simulink model "PlatooningUsingV2VTestBench"  (R2025a)
settings: Solver=ode23tb  StartTime=0.0  StopTime=stopTime  RelTol=1e-1  AbsTol=5e-5
PostLoadFcn:
  | helperSLPlatooningUsingV2VSetup
InitFcn:
  | figureName = 'Platooning Simulation Results';
  | hFig = findobj('Type','Figure','Name',figureName);
  | close(hFig)
values from neighbouring files (symbols this model uses):
  L = vehicleDimension.TractorLength + vehicleDimension.TrailerLength + vehicleDimension.InterConnection - vehicleDimension.Overlap + spacing    [helperSLPlatooningUsingV2VSetup.m]
  spacing = 7    [helperSLPlatooningUsingV2VSetup.m]
undefined symbols (not defined in the file or in its folder): accelerationProfile, C1, DiscIntNeverNeededParam, initialActorPose, K1, K2, N, sceneOrigin, Sim3dSensor, tractor, Ts, Tsv, vehicleDimension
libraries: simulink x7, sim3dautolib x6, slpidlib x2, sim3dcameralib x1, sim3dlib x1, visionsinks x1
(part 1 of 2)
CloseFcn:
  | helperSLPlatooningUsingV2VCleanup
settings Model: SimulationMode=accelerator  Creator=The MathWorks, Inc.  LastModifiedBy=The MathWorks, Inc.
settings SolverCC: SolverJacobianMethodControl=FullPerturbation  ZeroCrossAlgorithm=Adaptive  DecoupledContinuousIntegration=on  MinimalZcImpactIntegration=on  MaxZcPerStep=1.0
settings OptimizationCC: ReuseModelBlockBuffer=off
settings DebuggingCC: IgnoredZcDiagnostic=none  UnconnectedInputMsg=warning  UnconnectedOutputMsg=warning  UnconnectedLineMsg=warning  SubsystemReferenceDiagnosticForUnitTest=warning
settings ModelReferenceCC: EnableRefExpFcnMdlSchedulingChecks=on
settings RTWCC: GPUComputeCapability=3.5  DLArmComputeVersion=19.05

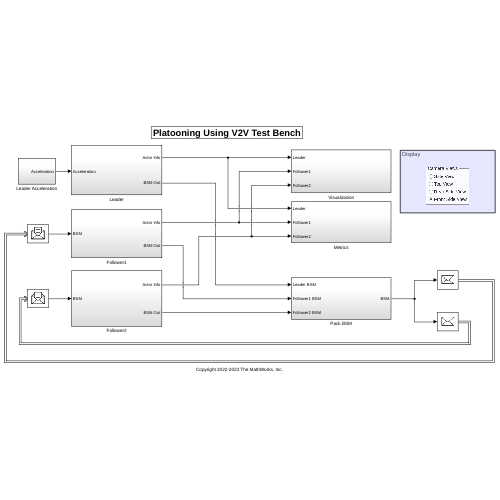
[thumbnail: Simulink's stored preview of the top-level diagram]
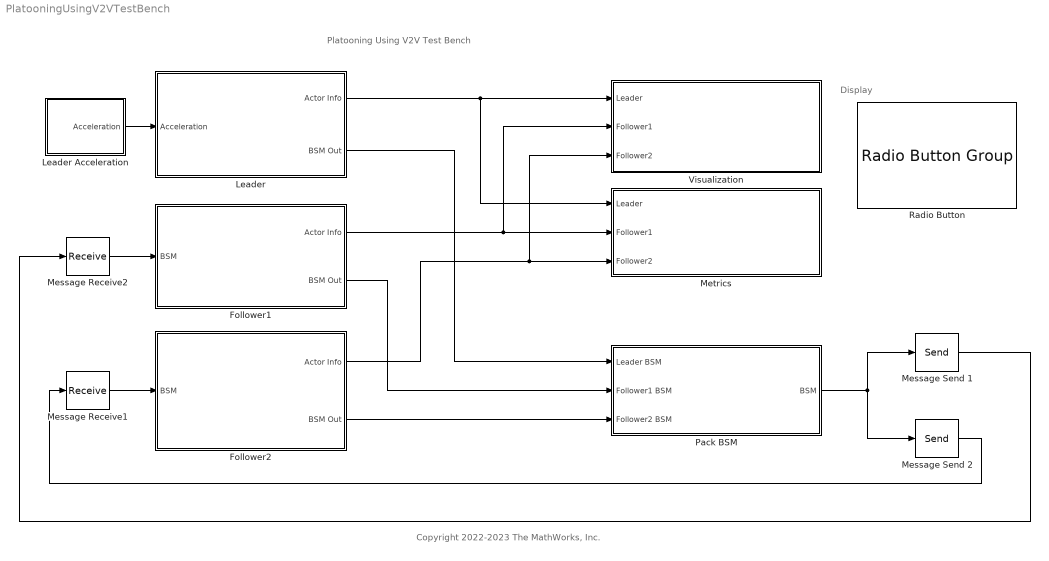
== system PlatooningUsingV2VTestBench ==
  note: Display
  note: Platooning Using V2V Test Bench
  note: Copyright 2022-2023 The MathWorks, Inc.
  Follower1 : Subsystem
  Follower2 : Subsystem
  Leader : Subsystem
  Leader Acceleration : Subsystem
  Message Receive1 : Receive  InputPortMessageModes=m  UseInternalQueue=off  SampleTime=Ts
  Message Receive2 : Receive  InputPortMessageModes=m  UseInternalQueue=off  SampleTime=Ts
  Message Send 1 : Send  OutputPortMessageModes=m
  Message Send 2 : Send  OutputPortMessageModes=m
  Metrics : Subsystem
  Pack BSM : Subsystem
  Radio Button : RadioButtonGroup  LabelPosition=Hide  SelectedLabel=Front Side View  ButtonGroupName=Camera Views
  Visualization : Subsystem
  wires:
  Leader Acceleration/1(Acceleration) -> Leader/1(Acceleration)
  Message Receive1/1 -> Follower2/1(BSM)
  Message Receive2/1 -> Follower1/1(BSM)
  Pack BSM/1(BSM) -> Message Send 2/1, Message Send 1/1
  Follower2/2(BSM Out) -> Pack BSM/3(Follower2 BSM)
  Follower1/2(BSM Out) -> Pack BSM/2(Follower1 BSM)
  Leader/2(BSM Out) -> Pack BSM/1(Leader BSM)
  Leader/1(Actor Info) -> Visualization/1(Leader), Metrics/1(Leader)
  Follower1/1(Actor Info) -> Metrics/2(Follower1), Visualization/2(Follower1)
  Follower2/1(Actor Info) -> Metrics/3(Follower2), Visualization/3(Follower2)
  Message Send 2/1 -> Message Receive1/1
  Message Send 1/1 -> Message Receive2/1

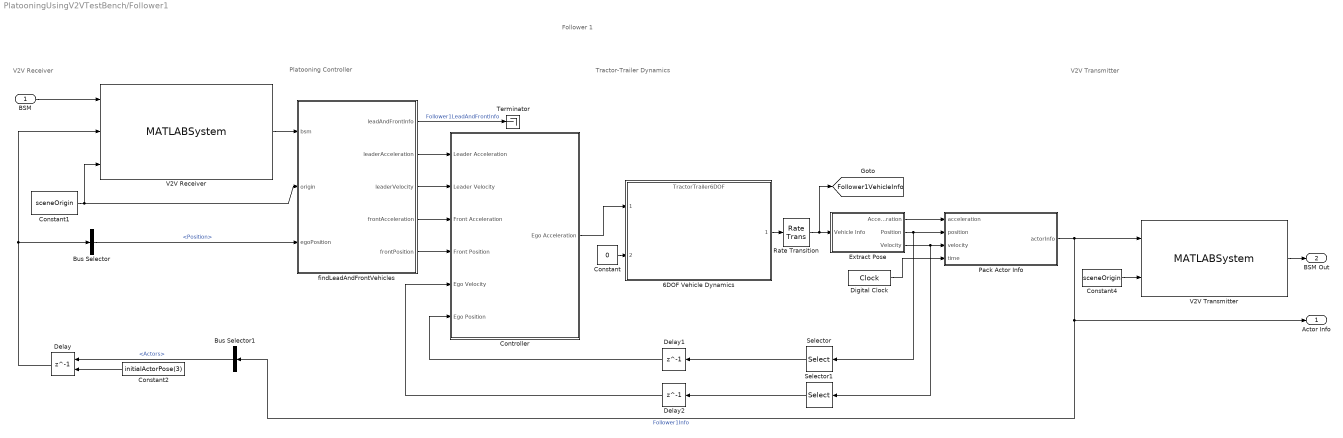
== system PlatooningUsingV2VTestBench/Follower1 ==
  note: V2V Transmitter
  note: Follower 1
  note: Tractor-Trailer Dynamics
  note: Platooning Controller
  note: V2V Receiver
  BSM : Inport
  6DOF Vehicle Dynamics : ModelReference  ModelNameDialog=TractorTrailer6DOF.slx  UsingDefaultArgumentValue=0,0,0,0,0,0,0,0  ModelReferenceVersion=5.2  initialTractorPosition=initialActorPose(3).Position  initialTractorVelocity=initialActorPose(3).Velocity  initialTractorOrientation=[0 0 0]  initialTractorRotationRates=[0 0 0]  initialTrailerPosition=initialActorPose(4).Position  initialTrailerVelocity=initialActorPose(4).Velocity  initialTrailerOrientation=[0 0 0]  initialTrailerRotationRates=[0 0 0]
  Bus Selector : BusSelector  OutputSignals=Position
  Bus Selector1 : BusSelector  OutputSignals=Actors
  Constant : Constant  Value=0  SampleTime=Ts
  Constant1 : Constant  Value=sceneOrigin  SampleTime=Ts
  Constant2 : Constant  Value=initialActorPose(3)  OutDataTypeStr=Bus: BusActorPose  SampleTime=-1
  Constant4 : Constant  Value=sceneOrigin  SampleTime=Ts
  Controller : Subsystem
  Delay : Delay  DelayLength=1  InitialConditionSource=Input port  SampleTime=Ts
      settings: InputPortMap=u0,p4
  Delay1 : Delay  DelayLength=1  InitialCondition=initialActorPose(3).Position(1)
  Delay2 : Delay  DelayLength=1  InitialCondition=initialActorPose(3).Velocity(1)
  Digital Clock : DigitalClock  SampleTime=Ts
  Extract Pose : Subsystem
  Pack Actor Info : MATLAB Function  TreatAsAtomicUnit=on  mask{initialActorInfo=initialActorPose(3), outputStruct=Simulink.Bus.createMATLABStruct('BusActorsInfo')}
      mask prompts: initialActorInfo "Initial Actor Info"; outputStruct "Output Struct"
  Rate Transition : RateTransition  OutPortSampleTime=Ts
  Selector : Selector  InputPortWidth=3  IndexOptions=Index vector (dialog)  Indices=1  OutputSizes=1
  Selector1 : Selector  InputPortWidth=3  IndexOptions=Index vector (dialog)  Indices=1  OutputSizes=1
  Terminator : Terminator
  V2V Receiver : MATLABSystem  System=HelperV2VReceiver  SnrCurves=channelAttributes  OutputStruct=Simulink.Bus.createMATLABStruct('BusBSM')  SimulateUsing=Code generation
      mask Type: HelperV2VReceiver
  V2V Transmitter : MATLABSystem  System=HelperV2VTransmitter  SampleTime=Ts  OutputStruct=Simulink.Bus.createMATLABStruct('BusBSM')  SimulateUsing=Code generation
      mask Type: HelperV2VTransmitter
  findLeadAndFrontVehicles : MATLAB Function  TreatAsAtomicUnit=on  mask(Process BSM data){egoID=initialActorPose(3).ActorID, outputStruct=Simulink.Bus.createMATLABStruct('BusLeadAndFrontInfo')}
      mask prompts: egoID "Actor ID"; outputStruct "Output Struct"
      mask help: Convert the BSM input data into physical values and generates object detection reports for the inputs to the multiObjectTracker
  Actor Info : Outport
  BSM Out : Outport  Port=2
  tag scope: Follower1VehicleInfo=global
  wires:
  Controller/1("Ego Acceleration ") -> 6DOF Vehicle Dynamics/1
  BSM/1 -> V2V Receiver/1
  Constant1/1 -> V2V Receiver/3, findLeadAndFrontVehicles/2(origin)
  Constant2/1 -> Delay/2
  Delay/1 -> Bus Selector/1, V2V Receiver/2
  V2V Receiver/1 -> findLeadAndFrontVehicles/1(bsm)
  Delay1/1 -> Controller/6("Ego Position ")
  Delay2/1 -> Controller/5("Ego Velocity ")
  6DOF Vehicle Dynamics/1 -> Rate Transition/1
  Bus Selector/1 -> findLeadAndFrontVehicles/3(egoPosition)  "<Position>"
  findLeadAndFrontVehicles/2(leaderAcceleration) -> Controller/1(Leader Acceleration)
  findLeadAndFrontVehicles/3(leaderVelocity) -> Controller/2("Leader Velocity ")
  findLeadAndFrontVehicles/4(frontAcceleration) -> Controller/3("Front Acceleration ")
  findLeadAndFrontVehicles/5(frontPosition) -> Controller/4("Front Position ")
  Constant/1 -> 6DOF Vehicle Dynamics/2
  Rate Transition/1 -> Extract Pose/1(Vehicle Info), [Follower1VehicleInfo]
  Extract Pose/1(Acceleration) -> Pack Actor Info/1(acceleration)
  Extract Pose/2(Position) -> Selector/1, Pack Actor Info/2(position)
  Extract Pose/3(Velocity) -> Selector1/1, Pack Actor Info/3(velocity)
  Selector/1 -> Delay1/1
  Selector1/1 -> Delay2/1
  findLeadAndFrontVehicles/1(leadAndFrontInfo) -> Terminator/1  "Follower1LeadAndFrontInfo"
  V2V Transmitter/1 -> BSM Out/1
  Constant4/1 -> V2V Transmitter/2
  Pack Actor Info/1(actorInfo) -> V2V Transmitter/1, Actor Info/1, Bus Selector1/1  "Follower1Info"
  Digital Clock/1 -> Pack Actor Info/4(time)
  Bus Selector1/1 -> Delay/1  "<Actors>"

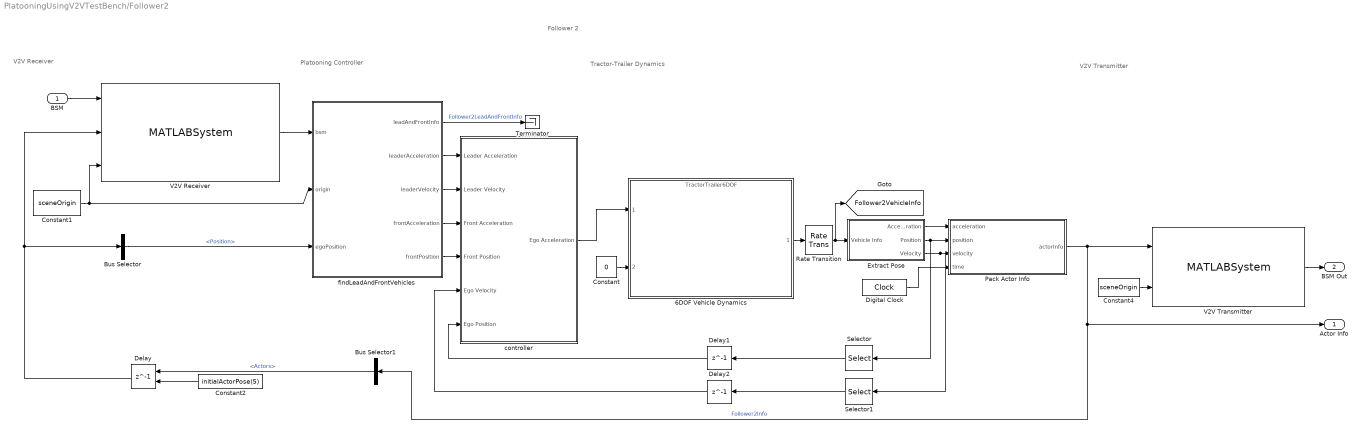
== system PlatooningUsingV2VTestBench/Follower2 ==
  note: V2V Receiver
  note: Follower 2
  note: Tractor-Trailer Dynamics
  note: Platooning Controller
  note: V2V Transmitter
  BSM : Inport
  6DOF Vehicle Dynamics : ModelReference  ModelNameDialog=TractorTrailer6DOF.slx  UsingDefaultArgumentValue=0,0,0,0,0,0,0,0  ModelReferenceVersion=5.2  initialTractorPosition=initialActorPose(5).Position  initialTractorVelocity=initialActorPose(5).Velocity  initialTractorOrientation=[0 0 0]  initialTractorRotationRates=[0 0 0]  initialTrailerPosition=initialActorPose(6).Position  initialTrailerVelocity=initialActorPose(6).Velocity  initialTrailerOrientation=[0 0 0]  initialTrailerRotationRates=[0 0 0]
  Bus Selector : BusSelector  OutputSignals=Position
  Bus Selector1 : BusSelector  OutputSignals=Actors
  Constant : Constant  Value=0  SampleTime=Ts
  Constant1 : Constant  Value=sceneOrigin  SampleTime=Ts
  Constant2 : Constant  Value=initialActorPose(5)  OutDataTypeStr=Bus: BusActorPose  SampleTime=-1
  Constant4 : Constant  Value=sceneOrigin  SampleTime=Ts
  Delay : Delay  DelayLength=1  InitialConditionSource=Input port  SampleTime=Ts
      settings: InputPortMap=u0,p4
  Delay1 : Delay  DelayLength=1  InitialCondition=initialActorPose(5).Position(1)
  Delay2 : Delay  DelayLength=1  InitialCondition=initialActorPose(5).Velocity(1)
  Digital Clock : DigitalClock  SampleTime=Ts
  Extract Pose : Subsystem
  Pack Actor Info : MATLAB Function  TreatAsAtomicUnit=on  mask{initialActorInfo=initialActorPose(5), outputStruct=Simulink.Bus.createMATLABStruct('BusActorsInfo')}
      mask prompts: initialActorInfo "Initial Actor Info"; outputStruct "Output Struct"
  Rate Transition : RateTransition  OutPortSampleTime=Ts
  Selector : Selector  InputPortWidth=3  IndexOptions=Index vector (dialog)  Indices=1  OutputSizes=1
  Selector1 : Selector  InputPortWidth=3  IndexOptions=Index vector (dialog)  Indices=1  OutputSizes=1
  Terminator : Terminator
  V2V Receiver : MATLABSystem  System=HelperV2VReceiver  SnrCurves=channelAttributes  OutputStruct=Simulink.Bus.createMATLABStruct('BusBSM')  SimulateUsing=Code generation
      mask Type: HelperV2VReceiver
  V2V Transmitter : MATLABSystem  System=HelperV2VTransmitter  SampleTime=Ts  OutputStruct=Simulink.Bus.createMATLABStruct('BusBSM')  SimulateUsing=Code generation
      mask Type: HelperV2VTransmitter
  controller : Subsystem
  findLeadAndFrontVehicles : MATLAB Function  TreatAsAtomicUnit=on  mask(Process BSM data){egoID=initialActorPose(5).ActorID, outputStruct=Simulink.Bus.createMATLABStruct('BusLeadAndFrontInfo')}
      mask prompts: egoID "Actor ID"; outputStruct "Output Struct"
      mask help: Convert the BSM input data into physical values and generates object detection reports for the inputs to the multiObjectTracker
  Actor Info : Outport
  BSM Out : Outport  Port=2
  tag scope: Follower2VehicleInfo=global
  wires:
  findLeadAndFrontVehicles/5(frontPosition) -> controller/4("Front Position ")
  findLeadAndFrontVehicles/3(leaderVelocity) -> controller/2(Leader Velocity)
  findLeadAndFrontVehicles/2(leaderAcceleration) -> controller/1(Leader Acceleration)
  BSM/1 -> V2V Receiver/1
  V2V Receiver/1 -> findLeadAndFrontVehicles/1(bsm)
  findLeadAndFrontVehicles/4(frontAcceleration) -> controller/3("Front Acceleration ")
  Constant1/1 -> V2V Receiver/3, findLeadAndFrontVehicles/2(origin)
  Constant2/1 -> Delay/2
  Delay/1 -> V2V Receiver/2, Bus Selector/1
  controller/1("Ego Acceleration ") -> 6DOF Vehicle Dynamics/1
  Delay1/1 -> controller/6(Ego Position)
  Delay2/1 -> controller/5("Ego Velocity ")
  6DOF Vehicle Dynamics/1 -> Rate Transition/1
  Bus Selector/1 -> findLeadAndFrontVehicles/3(egoPosition)  "<Position>"
  Extract Pose/1(Acceleration) -> Pack Actor Info/1(acceleration)
  Constant/1 -> 6DOF Vehicle Dynamics/2
  Rate Transition/1 -> Extract Pose/1(Vehicle Info), [Follower2VehicleInfo]
  Extract Pose/2(Position) -> Pack Actor Info/2(position), Selector/1
  Extract Pose/3(Velocity) -> Selector1/1, Pack Actor Info/3(velocity)
  Selector/1 -> Delay1/1
  Selector1/1 -> Delay2/1
  findLeadAndFrontVehicles/1(leadAndFrontInfo) -> Terminator/1  "Follower2LeadAndFrontInfo"
  Constant4/1 -> V2V Transmitter/2
  Pack Actor Info/1(actorInfo) -> V2V Transmitter/1, Actor Info/1, Bus Selector1/1  "Follower2Info"
  V2V Transmitter/1 -> BSM Out/1
  Digital Clock/1 -> Pack Actor Info/4(time)
  Bus Selector1/1 -> Delay/1  "<Actors>"

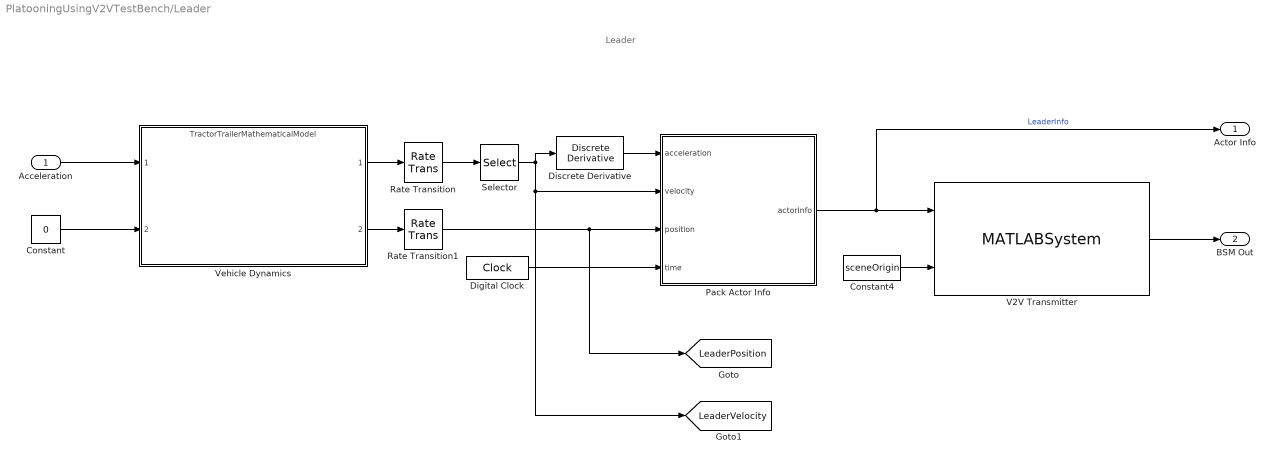
== system PlatooningUsingV2VTestBench/Leader ==
  note: Leader
  Acceleration : Inport
  Constant : Constant  Value=0
  Constant4 : Constant  Value=sceneOrigin  SampleTime=Ts
  Digital Clock : DigitalClock  SampleTime=Ts
  Discrete Derivative : simulink/Discrete/Discrete Derivative  gainval=1.0  ICPrevScaledInput=0.0  OutMin=[]  OutMax=[]  OutDataType=fixdt(1, 16)  OutScaling=2^-10  DoSatur=off
  Pack Actor Info : MATLAB Function  TreatAsAtomicUnit=on  mask{initialActorInfo=initialActorPose(1), outputStruct=Simulink.Bus.createMATLABStruct('BusActorsInfo')}
      mask prompts: initialActorInfo "Initial Actor Info"; outputStruct "Output Struct"
  Rate Transition : RateTransition  OutPortSampleTime=Ts
  Rate Transition1 : RateTransition  OutPortSampleTime=Ts
  Selector : Selector  InputPortWidth=8  IndexOptions=Index vector (dialog)  Indices=[1 2]  OutputSizes=1
  V2V Transmitter : MATLABSystem  System=HelperV2VTransmitter  SampleTime=Ts  OutputStruct=Simulink.Bus.createMATLABStruct('BusBSM')  SimulateUsing=Code generation
      mask Type: HelperV2VTransmitter
  Vehicle Dynamics : ModelReference  ModelNameDialog=TractorTrailerMathematicalModel.slx  UsingDefaultArgumentValue=0,0,0,0  SimulationMode=Normal  ModelReferenceVersion=3.0  initialPosition=initialActorPose(1).Position  initialVelocity=initialActorPose(1).Velocity  theta=0  beta=0
  Actor Info : Outport
  BSM Out : Outport  Port=2
  tag scope: LeaderPosition=global, LeaderVelocity=global
  wires:
  Vehicle Dynamics/1 -> Rate Transition/1
  Vehicle Dynamics/2 -> Rate Transition1/1
  Acceleration/1 -> Vehicle Dynamics/1
  Constant/1 -> Vehicle Dynamics/2
  Discrete Derivative/1 -> Pack Actor Info/1(acceleration)
  Rate Transition/1 -> Selector/1
  Rate Transition1/1 -> [LeaderPosition], Pack Actor Info/3(position)
  Selector/1 -> [LeaderVelocity], Pack Actor Info/2(velocity), Discrete Derivative/1
  Pack Actor Info/1(actorInfo) -> Actor Info/1, V2V Transmitter/1  "LeaderInfo"
  Constant4/1 -> V2V Transmitter/2
  V2V Transmitter/1 -> BSM Out/1
  Digital Clock/1 -> Pack Actor Info/4(time)

== system PlatooningUsingV2VTestBench/Leader Acceleration ==
  Pulse Generator : DiscretePulseGenerator  PulseType=Time based  Amplitude=accelerationProfile.Amplitude(1)  Period=accelerationProfile.Period  PulseWidth=accelerationProfile.PulseWidth(1)  PhaseDelay=accelerationProfile.PhaseDelay(1)
  Pulse Generator1 : DiscretePulseGenerator  PulseType=Time based  Amplitude=accelerationProfile.Amplitude(2)  Period=accelerationProfile.Period  PulseWidth=accelerationProfile.PulseWidth(2)  PhaseDelay=accelerationProfile.PhaseDelay(2)
  Rate Limiter : RateLimiter  RisingSlewLimit=0.5  FallingSlewLimit=-0.5  SampleTimeMode=inherited
  Sum : Sum
  Acceleration : Outport
  wires:
  Rate Limiter/1 -> Acceleration/1
  Pulse Generator/1 -> Sum/1
  Pulse Generator1/1 -> Sum/2
  Sum/1 -> Rate Limiter/1

== system PlatooningUsingV2VTestBench/Metrics ==
  note: Metrics Assessment
  Leader : Inport
  Follower1 : Inport  Port=2
  Follower2 : Inport  Port=3
  Collision Metrics : Subsystem
  Compute Spacing : MATLAB Function  TreatAsAtomicUnit=on  mask{expectedSpacing=L}
      mask prompts: expectedSpacing "Expected Spacing"
  Spacing Metrics : Subsystem
  wires:
  Leader/1 -> Compute Spacing/1(leader)
  Compute Spacing/2(spacing12) -> Collision Metrics/1(Spacing 1), Spacing Metrics/1(Spacing 1)
  Compute Spacing/3(spacing23) -> Spacing Metrics/2(Spacing 2), Collision Metrics/2(Spacing 2)
  Compute Spacing/1(isPlatoonFormed) -> Spacing Metrics/Enable
  Follower1/1 -> Compute Spacing/2(follower1)
  Follower2/1 -> Compute Spacing/3(follower2)

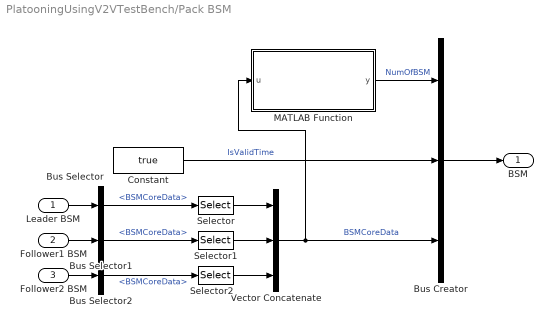
== system PlatooningUsingV2VTestBench/Pack BSM ==
  Leader BSM : Inport
  Follower1 BSM : Inport  Port=2
  Follower2 BSM : Inport  Port=3
  Bus Creator : BusCreator  Inputs=3  OutDataTypeStr=Bus: BusBSM  NonVirtualBus=on
  Bus Selector : BusSelector  OutputSignals=BSMCoreData
  Bus Selector1 : BusSelector  OutputSignals=BSMCoreData
  Bus Selector2 : BusSelector  OutputSignals=BSMCoreData
  Constant : Constant  Value=true
  MATLAB Function : MATLAB Function  TreatAsAtomicUnit=on
  Selector : Selector  InputPortWidth=3  IndexOptions=Index vector (dialog)  Indices=1  OutputSizes=1
  Selector1 : Selector  InputPortWidth=3  IndexOptions=Index vector (dialog)  Indices=1  OutputSizes=1
  Selector2 : Selector  InputPortWidth=3  IndexOptions=Index vector (dialog)  Indices=1  OutputSizes=1
  Vector Concatenate : Concatenate  NumInputs=3
  BSM : Outport
  wires:
  Constant/1 -> Bus Creator/2  "IsValidTime"
  MATLAB Function/1(y) -> Bus Creator/1  "NumOfBSM"
  Follower1 BSM/1 -> Bus Selector1/1
  Leader BSM/1 -> Bus Selector/1
  Vector Concatenate/1 -> Bus Creator/3, MATLAB Function/1(u)  "BSMCoreData"
  Bus Creator/1 -> BSM/1
  Follower2 BSM/1 -> Bus Selector2/1
  Bus Selector/1 -> Selector/1  "<BSMCoreData>"
  Bus Selector1/1 -> Selector1/1  "<BSMCoreData>"
  Bus Selector2/1 -> Selector2/1  "<BSMCoreData>"
  Selector/1 -> Vector Concatenate/1
  Selector2/1 -> Vector Concatenate/3
  Selector1/1 -> Vector Concatenate/2

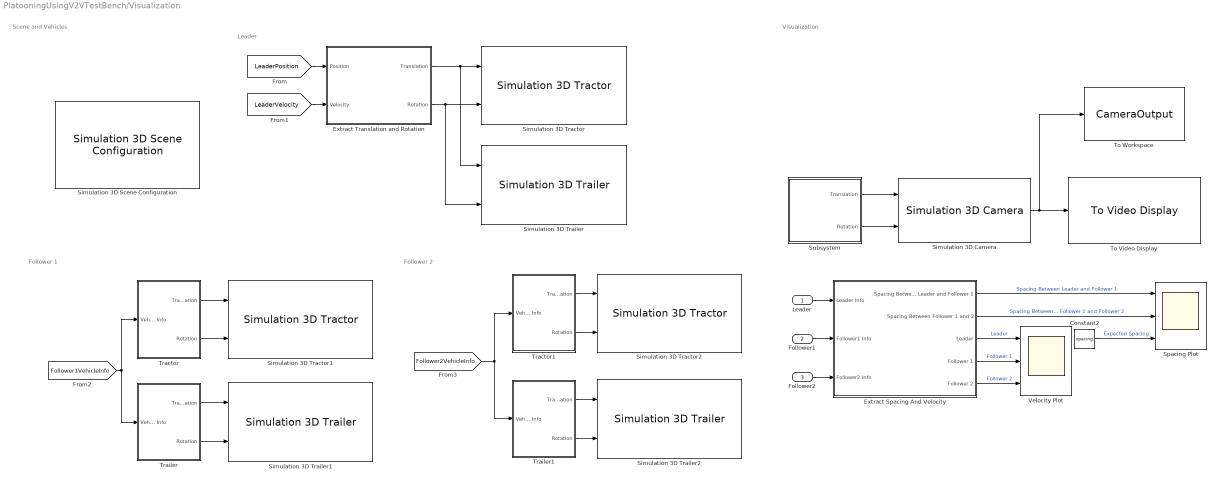
== system PlatooningUsingV2VTestBench/Visualization ==
  note: Follower 2
  note: Follower 1
  note: Leader
  note: Scene and Vehicles
  note: Visualization
  Leader : Inport  SampleTime=Tsv
  Follower1 : Inport  Port=2  SampleTime=Tsv
  Follower2 : Inport  Port=3  SampleTime=Tsv
  Constant2 : Constant  Value=spacing  SampleTime=Tsv
  Extract Spacing And Velocity : Subsystem
  "Extract Translation and Rotation " : Subsystem
  Simulation 3D Camera : sim3dcameralib/Simulation 3D Camera  Priority=1  sensorTag=Sim3dSensor�  sensorId=5  sensorName=Sim3dSensor�  vehTagList={'Follower1Tractor';'Follower1Trailer';'Follower2Tractor';'Follower2Trailer';'LeaderTractor';'LeaderTrailer';'Scene Origin'}  vehTag=Follower1Tractor  CoordinateSystem=ISO8855  mountLoc=Origin  offsetFlag=on  tmountOffset=initialCameraView.Translation  extTmount=on  rmountOffset=initialCameraView.Rotation  extRmount=on  FocalLength=[1000,1000]  OpticalCenter=[640, 360]  ImageSize=[720,1280]  RadialDistortion=[0, 0]  TangentialDistortion=[0, 0]  SensorSkew=0  VisualizeFieldOfView=off  FieldOfViewRange=61  DepthOutportEnabled=off  SemanticOutportEnabled=off  TransformOutportEnabled=off  SampleTime=Tsv  mountPoint=[100 85 85]  mountOrientation=[0 35 -135]  aMode=3  ID=5
      settings: LibrarySourceBlock=drivingsim3d/Simulation 3D Camera
  Simulation 3D Scene Configuration : sim3dlib/Simulation 3D Scene Configuration  Priority=0  ProjectFormat=Default Scenes  SceneDesc=Straight road  ProjectName=/mathworks/devel/bat/filer/batfs2566-0/Bdoc25a.2974004/build/runnable/matlab/toolbox/shared/sim3d_projects/automotive_project_linux/UE/LinuxNoEditor/VehicleSimulation.sh  ScenePath=/Game/Maps/HwStrght  EnableOpenDRIVE=off  vehTagList={'Follower1Tractor';'Follower1Trailer';'Follower2Tractor';'Follower2Trailer';'LeaderTractor';'LeaderTrailer';'Scene Origin'}  vehTag=LeaderTractor  AttachedCameraRelativeTranslation=[0 0 0]  FreeCameraDefaultInitialTranslation=[-6, 0, 2]  AttachedCameraRelativeRotation=[0 0 0]  FreeCameraDefaultInitialRotation=[0, -15, 0]  ViewpointName=Custom  FreeCameraInitialTranslation=[0 0 0]  ViewpointTranslation=[0 0 0]  FreeCameraInitialRotation=[0 0 0]  ViewpointRotation=[0 0 0]  OpVisEn=off  Ts=Tsv  EnableWindow=off  EnableRemoteAccess=off  EnableWeather=off  SunAzimuth=90  SunAltitude=40.0  EnableGeospatialSun=off  Latitude=0  Longitude=0  Date=2023-01-01  Time=10:30:00  GeoTimeZone=-5.0  SunDaylightSaving=off  wind=1  clouds=10  EnableVolumetricClouds=off  CloudCoverage=0  CloudAltitude=6  fog=0  rain=0  RaindropsEffect=off  SnowDensity=0  EnableGeospatial=off  TilesetSource=Earth terrain  UseTrueOrigin=off  OriginHeight=200  OriginLatitude=40.744652  OriginLongitude=-73.988864  MapStyle=Aerial  AdditionalAssetIDs=[]  UseAdvancedSunSky=off  SolarTime=11  TimeZone=-5  Day=21  Month=9  Year=2022  UseDaylightSavingTime=on  DSTStartDay=10  DSTStartMonth=3  DSTEndDay=3  DSTEndMonth=11  DSTSwitchHour=2  sensorTag=MainCamera1  sensorId=1  sensorName=MainCamera1  mountLoc=Origin  offsetFlag=off  tmountOffset=[0, 0, 0]  rmountOffset=[0, 0, 0]  HorizontalResolution=1280  VerticalResolution=720  HorizontalFOV=60  mountPoint=[0 0 0]  mountOrientation=[0 0 0]  aMode=2  ID=1  GeoTrigger=Inactive  ViewNameList={'Custom'}  ViewTranslationList={'[0 0 0]'}  ViewRotationList={'[0 0 0]'}
      settings: LibrarySourceBlock=vdynlib/Vehicle Scenarios/Sim3D/Sim3D Core/Simulation 3D Scene Configuration
  Simulation 3D Tractor : sim3dautolib/Simulation 3D Tractor  Priority=-1  Mesh=Cab-over tractor  TractorColor=Red  ActorName=LeaderTractor  Translation=[initialActorPose(1).Position;zeros( 6, 3 )]  Rotation=zeros( 7, 3 )  SampleTime=Tsv  ActorType=SimulinkVehicle  ID=C  aMode=2  ActorTag=LeaderTractor
      settings: LibrarySourceBlock=vdynlib/Vehicle Scenarios/Sim3D/Sim3D Vehicle/Components/Simulation 3D Tractor
  Simulation 3D Tractor1 : sim3dautolib/Simulation 3D Tractor  Priority=-1  Mesh=Cab-over tractor  TractorColor=Red  ActorName=Follower1Tractor  Translation=[initialActorPose(3).Position;zeros( 6, 3 )]  Rotation=zeros( 7, 3 )  SampleTime=Tsv  ActorType=SimulinkVehicle  ID=C  aMode=2  ActorTag=Follower1Tractor
      settings: LibrarySourceBlock=vdynlib/Vehicle Scenarios/Sim3D/Sim3D Vehicle/Components/Simulation 3D Tractor
  Simulation 3D Tractor2 : sim3dautolib/Simulation 3D Tractor  Priority=-1  Mesh=Cab-over tractor  TractorColor=Red  ActorName=Follower2Tractor  Translation=[initialActorPose(5).Position;zeros( 6, 3 )]  Rotation=zeros( 7, 3 )  SampleTime=Tsv  ActorType=SimulinkVehicle  ID=C  aMode=2  ActorTag=Follower2Tractor
      settings: LibrarySourceBlock=vdynlib/Vehicle Scenarios/Sim3D/Sim3D Vehicle/Components/Simulation 3D Tractor
  Simulation 3D Trailer : sim3dautolib/Simulation 3D Trailer  Priority=-1  Mesh=Three-axle trailer  ActorName=LeaderTrailer  Translation=[initialActorPose(1).Position;zeros( 6, 3 )]  Rotation=zeros(7,3)  SampleTime=Tsv  ActorType=SimulinkVehicle  ID=2  aMode=2  ActorTag=LeaderTrailer
      settings: LibrarySourceBlock=vdynlib/Vehicle Scenarios/Sim3D/Sim3D Vehicle/Components/Simulation 3D Trailer
  Simulation 3D Trailer1 : sim3dautolib/Simulation 3D Trailer  Priority=-1  Mesh=Three-axle trailer  ActorName=Follower1Trailer  Translation=[initialActorPose(3).Position;zeros( 6, 3 )]  Rotation=zeros(7,3)  SampleTime=Tsv  ActorType=SimulinkVehicle  ID=C  aMode=2  ActorTag=Follower1Trailer
      settings: LibrarySourceBlock=vdynlib/Vehicle Scenarios/Sim3D/Sim3D Vehicle/Components/Simulation 3D Trailer
  Simulation 3D Trailer2 : sim3dautolib/Simulation 3D Trailer  Priority=-1  Mesh=Three-axle trailer  ActorName=Follower2Trailer  Translation=[initialActorPose(5).Position;zeros( 6, 3 )]  Rotation=zeros(7,3)  SampleTime=Tsv  ActorType=SimulinkVehicle  ID=C  aMode=2  ActorTag=Follower2Trailer
      settings: LibrarySourceBlock=vdynlib/Vehicle Scenarios/Sim3D/Sim3D Vehicle/Components/Simulation 3D Trailer
  Spacing Plot : Scope  NumInputPorts=3
  Subsystem : Subsystem
  To Video Display : visionsinks/To Video Display  windowSizeMode=True size (1:1)  openAtMdlStart=on  fullScreen=off  videoWindowX=536805376  videoWindowY=536805376  saveWindowSize=off  videoWindowWidth=1280  videoWindowHeight=720  inputColorFormat=RGB  inputType=Obsolete  imagePorts=One multidimensional signal  OutputDevice=On-screen video monitor  dataOrg=Column-major  isWindowOpen=off
  To Workspace : ToWorkspace  VariableName=CameraOutput  SampleTime=-1
  Tractor : Subsystem
  Tractor1 : Subsystem
  Trailer : Subsystem
  Trailer1 : Subsystem
  Velocity Plot : Scope  NumInputPorts=3
  wires:
  Constant2/1 -> Spacing Plot/3  "Expected Spacing"
  Simulation 3D Camera/1 -> To Workspace/1, To Video Display/1
  Extract Spacing And Velocity/1(Spacing Between Leader and Follower 1) -> Spacing Plot/1  "Spacing Between Leader and Follower 1"
  Extract Spacing And Velocity/2(Spacing Between Follower 1 and 2) -> Spacing Plot/2  "Spacing Between Follower 1 and Follower 2"
  Extract Spacing And Velocity/3(Leader) -> Velocity Plot/1  "Leader"
  Extract Spacing And Velocity/4(Follower 1) -> Velocity Plot/2  "Follower 1"
  Extract Spacing And Velocity/5(Follower 2) -> Velocity Plot/3  "Follower 2"
  Tractor/1(Translation) -> Simulation 3D Tractor1/1
  Tractor/2(Rotation) -> Simulation 3D Tractor1/2
  Trailer/1(Translation) -> Simulation 3D Trailer1/1
  Trailer/2(Rotation) -> Simulation 3D Trailer1/2
  Tractor1/1(Translation) -> Simulation 3D Tractor2/1
  Tractor1/2(Rotation) -> Simulation 3D Tractor2/2
  Trailer1/1(Translation) -> Simulation 3D Trailer2/1
  Trailer1/2(Rotation) -> Simulation 3D Trailer2/2
  [Follower1VehicleInfo] -> Tractor/1(Vehicle Info), Trailer/1(Vehicle Info)
  [Follower2VehicleInfo] -> Trailer1/1(Vehicle Info), Tractor1/1(Vehicle Info)
  "Extract Translation and Rotation "/1(Translation) -> Simulation 3D Tractor/1, Simulation 3D Trailer/1
  "Extract Translation and Rotation "/2(Rotation) -> Simulation 3D Tractor/2, Simulation 3D Trailer/2
  [LeaderVelocity] -> "Extract Translation and Rotation "/2(Velocity)
  [LeaderPosition] -> "Extract Translation and Rotation "/1(Position)
  Subsystem/1(Translation) -> Simulation 3D Camera/1
  Subsystem/2(Rotation) -> Simulation 3D Camera/2
  Leader/1 -> Extract Spacing And Velocity/1(Leader Info)
  Follower1/1 -> Extract Spacing And Velocity/2(Follower1 Info)
  Follower2/1 -> Extract Spacing And Velocity/3(Follower2 Info)

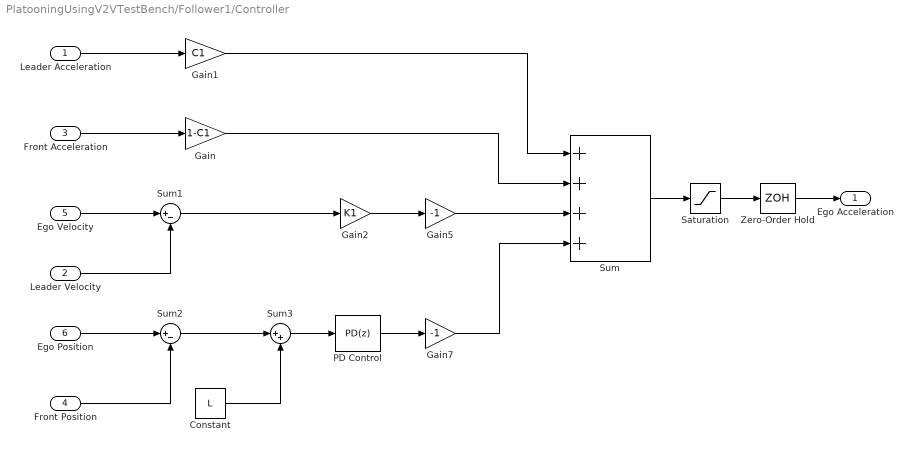
== system PlatooningUsingV2VTestBench/Follower1/Controller ==
  Leader Acceleration : Inport
  "Leader Velocity " : Inport  Port=2
  "Front Acceleration " : Inport  Port=3
  "Front Position " : Inport  Port=4
  "Ego Velocity " : Inport  Port=5
  "Ego Position " : Inport  Port=6
  Constant : Constant  Value=L  SampleTime=-1
  Gain : Gain  Gain=1-C1
  Gain1 : Gain  Gain=C1
  Gain2 : Gain  Gain=K1
  Gain5 : Gain  Gain=-1
  Gain7 : Gain  Gain=-1
  PD Control : slpidlib/PID Controller  Controller=PD  Form=Parallel  TimeDomain=Discrete-time  UseExternalTs=off  SampleTime=Ts  IntegratorMethod=Forward Euler  FilterMethod=Forward Euler  ControllerParametersSource=internal  P=K2(1)  I=K2(2)  UseKiTs=off  D=K2(2)  UseExternalDerivativeSource=off  N=N  UseFilter=on  TunerSelectOption=Frequency Response Based  ZeroCross=off  InitialConditionSource=internal  InitialConditionForIntegrator=0  InitialConditionForFilter=0  DifferentiatorICPrevScaledInput=0  ExternalReset=none  TrackingMode=off  Kt=1  LimitOutput=off  SatLimitsSource=internal  UpperSaturationLimit=inf  LowerSaturationLimit=-inf  LinearizeAsGain=on  AntiWindupMode=none  Kb=1  LimitIntegrator=off  UpperIntegratorSaturationLimit=inf  LowerIntegratorSaturationLimit=-inf  POutMin=[]  POutMax=[]  IOutMin=[]  IOutMax=[]  DOutMin=[]  DOutMax=[]  NOutMin=[]  NOutMax=[]  SumOutMin=[]  SumOutMax=[]  SaturationOutMin=[]  SaturationOutMax=[]  PParamMin=[]  PParamMax=[]  IParamMin=[]  IParamMax=[]  DParamMin=[]  DParamMax=[]  NParamMin=[]  NParamMax=[]  KbParamMin=[]  KbParamMax=[]  KtParamMin=[]  KtParamMax=[]  KbOutMin=[]  KbOutMax=[]  KtOutMin=[]  KtOutMax=[]  IntegratorOutMin=[]  IntegratorOutMax=[]  FilterOutMin=[]  FilterOutMax=[]  SumI1OutMin=[]  SumI1OutMax=[]  SumI2OutMin=[]  SumI2OutMax=[]  SumI3OutMin=[]  SumI3OutMax=[]  SumI4OutMin=[]  SumI4OutMax=[]  SumDOutMin=[]  SumDOutMax=[]  DifferentiatorOutMin=[]  DifferentiatorOutMax=[]  FilterDiffOutCoefMin=[]  FilterDiffOutCoefMax=[]  ReciprocalOutMin=[]  ReciprocalOutMax=[]  SumDenOutMin=[]  SumDenOutMax=[]  SumNumOutMin=[]  SumNumOutMax=[]  DivideOutMin=[]  DivideOutMax=[]  UdiffTsProdOutMin=[]  UdiffTsProdOutMax=[]  NTsProdOutMin=[]  NTsProdOutMax=[]  UintegralTsProdOutMin=[]  UintegralTsProdOutMax=[]  UngainTsProdOutMin=[]  UngainTsProdOutMax=[]  ClampingZeroOutDataTypeStr=Inherit: Inherit via back propagation  ClampingZeroOutMin=[]  ClampingZeroOutMax=[]  FilterDenConstantOutDataTypeStr=Inherit: Inherit via back propagation  FilterDenConstantOutMin=[]  FilterDenConstantOutMax=[]  PCopyOutDataTypeStr=Inherit: Inherit via back propagation  PCopyOutMin=[]  PCopyOutMax=[]  NCopyOutDataTypeStr=Inherit: Inherit via back propagation  NCopyOutMin=[]  NCopyOutMax=[]  IntegratorContinuousStateAttributes=''  IntegratorStateMustResolveToSignalObject=off  IntegratorRTWStateStorageClass=Auto  FilterContinuousStateAttributes=''  FilterStateMustResolveToSignalObject=off  FilterRTWStateStorageClass=Auto  ParallelPVariant=InternalParameters  IdealPVariant=Disabled  IVariant=Disabled  DVariant=InternalParameters  IntegratorVariant=Disabled  SatVariant=Disabled  AWVariant=Disabled  PCopyVariant=Disabled  TRVariant=Disabled  FdbkBlocksVariant=Forward  IdealPFdbkVariant=Disabled  SatFdbkVariant=Disabled  DerivativeFilterVariant=ForwardEulerFilter  NVariant=InternalParameters  NCopyVariant=Disabled  FilterICVariant=InternalICsFilter  IntegratorICVariant=Disabled  ExternalResetVariant=Disabled  TRSumVariant=Passthrough  SumFdbkVariant=Disabled  SumVariant=Sum_PD  TsampFilterVariant=InternalTs  TsampNgainVariant=Passthrough  TsampIntegralVariant=Disabled_SignalSpec  ExternalSaturationOutDataTypeStr=Inherit: Same as second input  DerivativeSourceVariant=ErrorSignal  PreIntVariant=InternalPreInt
  Saturation : Saturate  UpperLimit=3  LowerLimit=-5  ZeroCross=off
  Sum : Sum  Inputs=++++
  Sum1 : Sum  Inputs=|+-
  Sum2 : Sum  Inputs=|+-
  Sum3 : Sum  Inputs=|++
  Zero-Order Hold : ZeroOrderHold  SampleTime=-1
  "Ego Acceleration " : Outport
  wires:
  "Front Acceleration "/1 -> Gain/1
  Leader Acceleration/1 -> Gain1/1
  "Leader Velocity "/1 -> Sum1/2
  Sum1/1 -> Gain2/1
  Gain2/1 -> Gain5/1
  "Ego Position "/1 -> Sum2/1
  "Front Position "/1 -> Sum2/2
  Sum2/1 -> Sum3/1
  Constant/1 -> Sum3/2
  Gain7/1 -> Sum/4
  Gain/1 -> Sum/2
  Gain1/1 -> Sum/1
  "Ego Velocity "/1 -> Sum1/1
  Gain5/1 -> Sum/3
  Sum/1 -> Saturation/1
  Saturation/1 -> Zero-Order Hold/1
  Zero-Order Hold/1 -> "Ego Acceleration "/1
  PD Control/1 -> Gain7/1
  Sum3/1 -> PD Control/1

== system PlatooningUsingV2VTestBench/Follower1/Extract Pose ==
  Vehicle Info : Inport
  Bus Selector1 : BusSelector  OutputSignals=Tractor.Vehicle.InertFrm.Cg.Disp.X,Tractor.Vehicle.InertFrm.Cg.Disp.Y,Tractor.Vehicle.InertFrm.Cg.Disp.Z,Tractor.Vehicle.InertFrm.Cg.Vel.Xdot,Tractor.Vehicle.InertFrm.Cg.Vel.Ydot,Tractor.Vehicle.InertFrm.Cg.Vel.Zdot
  Discrete Derivative : simulink/Discrete/Discrete Derivative  gainval=1.0  ICPrevScaledInput=0.0  OutMin=[]  OutMax=[]  OutDataType=fixdt(1, 16)  OutScaling=2^-10  DoSatur=off
  Vector Concatenate : Concatenate  NumInputs=3
  Vector Concatenate1 : Concatenate  NumInputs=3
  Acceleration : Outport
  Position : Outport  Port=2
  Velocity : Outport  Port=3
  wires:
  Bus Selector1/2 -> Vector Concatenate/2  "<Y>"
  Vector Concatenate/1 -> Position/1
  Bus Selector1/1 -> Vector Concatenate/1  "<X>"
  Vehicle Info/1 -> Bus Selector1/1
  Bus Selector1/3 -> Vector Concatenate/3  "<Z>"
  Bus Selector1/4 -> Vector Concatenate1/1  "<Xdot>"
  Bus Selector1/5 -> Vector Concatenate1/2  "<Ydot>"
  Bus Selector1/6 -> Vector Concatenate1/3  "<Zdot>"
  Vector Concatenate1/1 -> Discrete Derivative/1, Velocity/1
  Discrete Derivative/1 -> Acceleration/1

== system PlatooningUsingV2VTestBench/Follower2/Extract Pose ==
  Vehicle Info : Inport
  Bus Selector1 : BusSelector  OutputSignals=Tractor.Vehicle.InertFrm.Cg.Disp.X,Tractor.Vehicle.InertFrm.Cg.Disp.Y,Tractor.Vehicle.InertFrm.Cg.Disp.Z,Tractor.Vehicle.InertFrm.Cg.Vel.Xdot,Tractor.Vehicle.InertFrm.Cg.Vel.Ydot,Tractor.Vehicle.InertFrm.Cg.Vel.Zdot
  Discrete Derivative : simulink/Discrete/Discrete Derivative  gainval=1.0  ICPrevScaledInput=0.0  OutMin=[]  OutMax=[]  OutDataType=fixdt(1, 16)  OutScaling=2^-10  DoSatur=off
  Vector Concatenate : Concatenate  NumInputs=3
  Vector Concatenate1 : Concatenate  NumInputs=3
  Acceleration : Outport
  Position : Outport  Port=2
  Velocity : Outport  Port=3
  wires:
  Bus Selector1/2 -> Vector Concatenate/2  "<Y>"
  Vector Concatenate/1 -> Position/1
  Bus Selector1/1 -> Vector Concatenate/1  "<X>"
  Vehicle Info/1 -> Bus Selector1/1
  Bus Selector1/3 -> Vector Concatenate/3  "<Z>"
  Bus Selector1/4 -> Vector Concatenate1/1  "<Xdot>"
  Bus Selector1/5 -> Vector Concatenate1/2  "<Ydot>"
  Bus Selector1/6 -> Vector Concatenate1/3  "<Zdot>"
  Vector Concatenate1/1 -> Discrete Derivative/1, Velocity/1
  Discrete Derivative/1 -> Acceleration/1

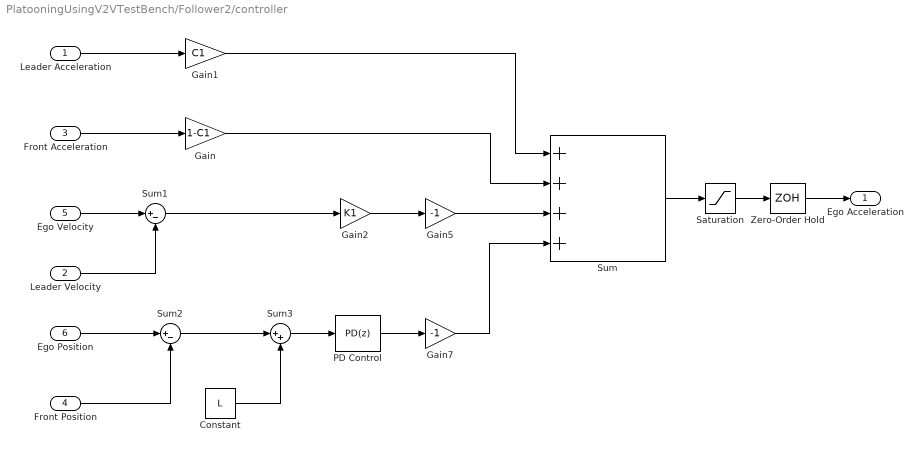
== system PlatooningUsingV2VTestBench/Follower2/controller ==
  Leader Acceleration : Inport
  Leader Velocity : Inport  Port=2
  "Front Acceleration " : Inport  Port=3
  "Front Position " : Inport  Port=4
  "Ego Velocity " : Inport  Port=5
  Ego Position : Inport  Port=6
  Constant : Constant  Value=L  SampleTime=-1
  Gain : Gain  Gain=1-C1
  Gain1 : Gain  Gain=C1
  Gain2 : Gain  Gain=K1
  Gain5 : Gain  Gain=-1
  Gain7 : Gain  Gain=-1
  PD Control : slpidlib/PID Controller  Controller=PD  Form=Parallel  TimeDomain=Discrete-time  UseExternalTs=off  SampleTime=Ts  IntegratorMethod=Forward Euler  FilterMethod=Forward Euler  ControllerParametersSource=internal  P=K2(1)  I=K2(2)  UseKiTs=off  D=K2(2)  UseExternalDerivativeSource=off  N=N  UseFilter=on  TunerSelectOption=Frequency Response Based  ZeroCross=off  InitialConditionSource=internal  InitialConditionForIntegrator=0  InitialConditionForFilter=0  DifferentiatorICPrevScaledInput=0  ExternalReset=none  TrackingMode=off  Kt=1  LimitOutput=off  SatLimitsSource=internal  UpperSaturationLimit=inf  LowerSaturationLimit=-inf  LinearizeAsGain=on  AntiWindupMode=none  Kb=1  LimitIntegrator=off  UpperIntegratorSaturationLimit=inf  LowerIntegratorSaturationLimit=-inf  POutMin=[]  POutMax=[]  IOutMin=[]  IOutMax=[]  DOutMin=[]  DOutMax=[]  NOutMin=[]  NOutMax=[]  SumOutMin=[]  SumOutMax=[]  SaturationOutMin=[]  SaturationOutMax=[]  PParamMin=[]  PParamMax=[]  IParamMin=[]  IParamMax=[]  DParamMin=[]  DParamMax=[]  NParamMin=[]  NParamMax=[]  KbParamMin=[]  KbParamMax=[]  KtParamMin=[]  KtParamMax=[]  KbOutMin=[]  KbOutMax=[]  KtOutMin=[]  KtOutMax=[]  IntegratorOutMin=[]  IntegratorOutMax=[]  FilterOutMin=[]  FilterOutMax=[]  SumI1OutMin=[]  SumI1OutMax=[]  SumI2OutMin=[]  SumI2OutMax=[]  SumI3OutMin=[]  SumI3OutMax=[]  SumI4OutMin=[]  SumI4OutMax=[]  SumDOutMin=[]  SumDOutMax=[]  DifferentiatorOutMin=[]  DifferentiatorOutMax=[]  FilterDiffOutCoefMin=[]  FilterDiffOutCoefMax=[]  ReciprocalOutMin=[]  ReciprocalOutMax=[]  SumDenOutMin=[]  SumDenOutMax=[]  SumNumOutMin=[]  SumNumOutMax=[]  DivideOutMin=[]  DivideOutMax=[]  UdiffTsProdOutMin=[]  UdiffTsProdOutMax=[]  NTsProdOutMin=[]  NTsProdOutMax=[]  UintegralTsProdOutMin=[]  UintegralTsProdOutMax=[]  UngainTsProdOutMin=[]  UngainTsProdOutMax=[]  ClampingZeroOutDataTypeStr=Inherit: Inherit via back propagation  ClampingZeroOutMin=[]  ClampingZeroOutMax=[]  FilterDenConstantOutDataTypeStr=Inherit: Inherit via back propagation  FilterDenConstantOutMin=[]  FilterDenConstantOutMax=[]  PCopyOutDataTypeStr=Inherit: Inherit via back propagation  PCopyOutMin=[]  PCopyOutMax=[]  NCopyOutDataTypeStr=Inherit: Inherit via back propagation  NCopyOutMin=[]  NCopyOutMax=[]  IntegratorContinuousStateAttributes=''  IntegratorStateMustResolveToSignalObject=off  IntegratorRTWStateStorageClass=Auto  FilterContinuousStateAttributes=''  FilterStateMustResolveToSignalObject=off  FilterRTWStateStorageClass=Auto  ParallelPVariant=InternalParameters  IdealPVariant=Disabled  IVariant=Disabled  DVariant=InternalParameters  IntegratorVariant=Disabled  SatVariant=Disabled  AWVariant=Disabled  PCopyVariant=Disabled  TRVariant=Disabled  FdbkBlocksVariant=Forward  IdealPFdbkVariant=Disabled  SatFdbkVariant=Disabled  DerivativeFilterVariant=ForwardEulerFilter  NVariant=InternalParameters  NCopyVariant=Disabled  FilterICVariant=InternalICsFilter  IntegratorICVariant=Disabled  ExternalResetVariant=Disabled  TRSumVariant=Passthrough  SumFdbkVariant=Disabled  SumVariant=Sum_PD  TsampFilterVariant=InternalTs  TsampNgainVariant=Passthrough  TsampIntegralVariant=Disabled_SignalSpec  ExternalSaturationOutDataTypeStr=Inherit: Same as second input  DerivativeSourceVariant=ErrorSignal  PreIntVariant=InternalPreInt
  Saturation : Saturate  UpperLimit=3  LowerLimit=-5  ZeroCross=off
  Sum : Sum  Inputs=++++
  Sum1 : Sum  Inputs=|+-
  Sum2 : Sum  Inputs=|+-
  Sum3 : Sum  Inputs=|++
  Zero-Order Hold : ZeroOrderHold  SampleTime=-1
  "Ego Acceleration " : Outport
  wires:
  "Front Acceleration "/1 -> Gain/1
  Leader Acceleration/1 -> Gain1/1
  Leader Velocity/1 -> Sum1/2
  Sum1/1 -> Gain2/1
  Gain2/1 -> Gain5/1
  Ego Position/1 -> Sum2/1
  "Front Position "/1 -> Sum2/2
  Sum2/1 -> Sum3/1
  Constant/1 -> Sum3/2
  Gain7/1 -> Sum/4
  Gain/1 -> Sum/2
  Gain1/1 -> Sum/1
  "Ego Velocity "/1 -> Sum1/1
  Gain5/1 -> Sum/3
  Sum/1 -> Saturation/1
  Saturation/1 -> Zero-Order Hold/1
  Zero-Order Hold/1 -> "Ego Acceleration "/1
  PD Control/1 -> Gain7/1
  Sum3/1 -> PD Control/1

== system PlatooningUsingV2VTestBench/Metrics/Collision Metrics ==
  Spacing 1 : Inport
  Spacing 2 : Inport  Port=2
  Check Static Lower Bound : simulink/Model Verification/Check Static  Lower Bound  Description=0 <= u  min=0  min_included=on  enabled=on  stopWhenAssertionFail=on  export=off  icon=graphic
  Check Static Lower Bound1 : simulink/Model Verification/Check Static  Lower Bound  Description=0 <= u  min=0  min_included=on  enabled=on  stopWhenAssertionFail=on  export=off  icon=graphic
  Constant : Constant  Value=L - spacing
  Sum : Sum  Inputs=|+-
  Sum1 : Sum  Inputs=|+-
  wires:
  Spacing 1/1 -> Sum/1
  Sum/1 -> Check Static Lower Bound/1
  Spacing 2/1 -> Sum1/1
  Constant/1 -> Sum/2, Sum1/2
  Sum1/1 -> Check Static Lower Bound1/1

== system PlatooningUsingV2VTestBench/Metrics/Spacing Metrics ==
  Spacing 1 : Inport
  Spacing 2 : Inport  Port=2
  Enable : EnablePort
  Check Static Range : simulink/Model Verification/Check  Static Range  Description=L-5 <= u <= L+5  max=L+5  max_included=on  min=L-5  min_included=on  enabled=on  stopWhenAssertionFail=off  export=off  icon=graphic
  Check Static Range1 : simulink/Model Verification/Check  Static Range  Description=L-5 <= u <= L+5  max=L+5  max_included=on  min=L-5  min_included=on  enabled=on  stopWhenAssertionFail=on  export=off  icon=graphic
  wires:
  Spacing 1/1 -> Check Static Range/1
  Spacing 2/1 -> Check Static Range1/1

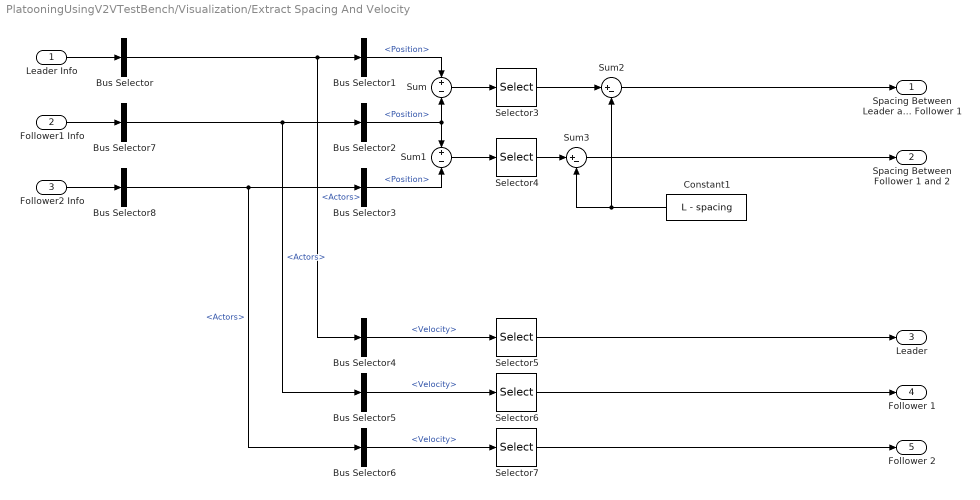
== system PlatooningUsingV2VTestBench/Visualization/Extract Spacing And Velocity ==
  Leader Info : Inport
  Follower1 Info : Inport  Port=2
  Follower2 Info : Inport  Port=3
  Bus Selector : BusSelector  OutputSignals=Actors
  Bus Selector1 : BusSelector  OutputSignals=Position
  Bus Selector2 : BusSelector  OutputSignals=Position
  Bus Selector3 : BusSelector  OutputSignals=Position
  Bus Selector4 : BusSelector  OutputSignals=Velocity
  Bus Selector5 : BusSelector  OutputSignals=Velocity
  Bus Selector6 : BusSelector  OutputSignals=Velocity
  Bus Selector7 : BusSelector  OutputSignals=Actors
  Bus Selector8 : BusSelector  OutputSignals=Actors
  Constant1 : Constant  Value=L - spacing
  Selector{3..7} (5 alike) : Selector  InputPortWidth=3  IndexOptions=Index vector (dialog)  Indices=1  OutputSizes=1
  Sum : Sum  Inputs=+-
  Sum1 : Sum  Inputs=+-
  Sum2 : Sum  Inputs=|+-
  Sum3 : Sum  Inputs=|+-
  Spacing Between Leader and Follower 1 : Outport
  Spacing Between Follower 1 and 2 : Outport  Port=2
  Leader : Outport  Port=3
  Follower 1 : Outport  Port=4
  Follower 2 : Outport  Port=5
  wires:
  Selector6/1 -> Follower 1/1
  Bus Selector1/1 -> Sum/1  "<Position>"
  Bus Selector/1 -> Bus Selector1/1, Bus Selector4/1  "<Actors>"
  Selector4/1 -> Sum3/1
  Bus Selector3/1 -> Sum1/2  "<Position>"
  Bus Selector2/1 -> Sum1/1, Sum/2  "<Position>"
  Sum3/1 -> Spacing Between Follower 1 and 2/1
  Sum/1 -> Selector3/1
  Sum1/1 -> Selector4/1
  Selector7/1 -> Follower 2/1
  Constant1/1 -> Sum3/2, Sum2/2
  Selector5/1 -> Leader/1
  Selector3/1 -> Sum2/1
  Leader Info/1 -> Bus Selector/1
  Bus Selector5/1 -> Selector6/1  "<Velocity>"
  Bus Selector6/1 -> Selector7/1  "<Velocity>"
  Bus Selector4/1 -> Selector5/1  "<Velocity>"
  Sum2/1 -> Spacing Between Leader and Follower 1/1
  Bus Selector7/1 -> Bus Selector2/1, Bus Selector5/1  "<Actors>"
  Bus Selector8/1 -> Bus Selector6/1, Bus Selector3/1  "<Actors>"
  Follower2 Info/1 -> Bus Selector8/1
  Follower1 Info/1 -> Bus Selector7/1

== system PlatooningUsingV2VTestBench/Visualization/Extract Translation and Rotation  ==
  Position : Inport
  Velocity : Inport  Port=2
  Constant1 : Constant  Value=vehicleDimension.TireRadius  SampleTime=Ts
  Discrete-Time Integrator : DiscreteIntegrator  SampleTime=-1  ICPrevOutput=DiscIntNeverNeededParam  ICPrevScaledInput=DiscIntNeverNeededParam
  Divide : Product  Inputs=*/
  Get Rotation : MATLAB Function  TreatAsAtomicUnit=on
  Get Translation : Subsystem
  Selector : Selector  InputPortWidth=2  IndexOptions=Index vector (dialog)  Indices=1  OutputSizes=1
  Translation : Outport
  Rotation : Outport  Port=2
  wires:
  Velocity/1 -> Selector/1
  Discrete-Time Integrator/1 -> Get Rotation/1(angularPos)
  Constant1/1 -> Divide/2
  Position/1 -> Get Translation/1(Position)
  Divide/1 -> Discrete-Time Integrator/1
  Get Translation/1(Translation) -> Translation/1
  Get Rotation/1(rotation) -> Rotation/1
  Selector/1 -> Divide/1

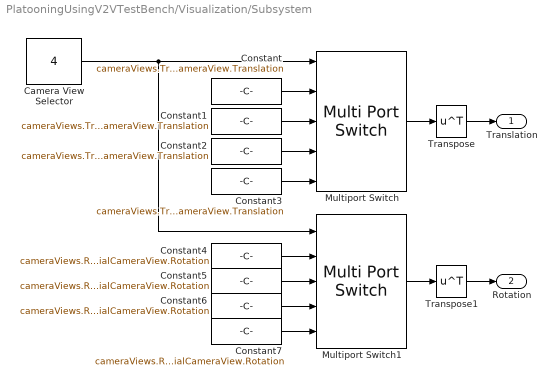
== system PlatooningUsingV2VTestBench/Visualization/Subsystem ==
  Camera View Selector : Constant  Value=4
  Constant : Constant  Value=cameraViews.Translation.SideView-initialCameraView.Translation
  Constant1 : Constant  Value=cameraViews.Translation.TopView-initialCameraView.Translation
  Constant2 : Constant  Value=cameraViews.Translation.RearSideView-initialCameraView.Translation
  Constant3 : Constant  Value=cameraViews.Translation.FrontSideView-initialCameraView.Translation
  Constant4 : Constant  Value=cameraViews.Rotation.SideView-initialCameraView.Rotation
  Constant5 : Constant  Value=cameraViews.Rotation.TopView-initialCameraView.Rotation
  Constant6 : Constant  Value=cameraViews.Rotation.RearSideView-initialCameraView.Rotation
  Constant7 : Constant  Value=cameraViews.Rotation.FrontSideView-initialCameraView.Rotation
  Multiport Switch : MultiPortSwitch  Inputs=4  SaturateOnIntegerOverflow=off  InputSameDT=off
  Multiport Switch1 : MultiPortSwitch  Inputs=4  SaturateOnIntegerOverflow=off  InputSameDT=off
  Transpose : Math  Operator=transpose
  Transpose1 : Math  Operator=transpose
  Translation : Outport
  Rotation : Outport  Port=2
  wires:
  Multiport Switch/1 -> Transpose/1
  Multiport Switch1/1 -> Transpose1/1
  Constant/1 -> Multiport Switch/2
  Constant1/1 -> Multiport Switch/3
  Constant2/1 -> Multiport Switch/4
  Constant3/1 -> Multiport Switch/5
  Constant7/1 -> Multiport Switch1/5
  Constant5/1 -> Multiport Switch1/3
  Constant4/1 -> Multiport Switch1/2
  Constant6/1 -> Multiport Switch1/4
  Camera View Selector/1 -> Multiport Switch1/1, Multiport Switch/1
  Transpose/1 -> Translation/1
  Transpose1/1 -> Rotation/1

== system PlatooningUsingV2VTestBench/Visualization/Tractor ==
  Vehicle Info : Inport
  Bus Selector : BusSelector  OutputSignals=Tractor
  Extract Tractor Rotation : Subsystem
  Extract Tractor Translation : Subsystem
  Translation : Outport
  Rotation : Outport  Port=2
  wires:
  Bus Selector/1 -> Extract Tractor Translation/1(Tractor), Extract Tractor Rotation/1(Tractor)  "<Tractor>"
  Extract Tractor Translation/1(Translation) -> Translation/1
  Vehicle Info/1 -> Bus Selector/1
  Extract Tractor Rotation/1(Rotation) -> Rotation/1

== system PlatooningUsingV2VTestBench/Visualization/Tractor1 ==
  Vehicle Info : Inport
  Bus Selector : BusSelector  OutputSignals=Tractor
  Extract Tractor Rotation : Subsystem
  Extract Tractor Translation : Subsystem
  Translation : Outport
  Rotation : Outport  Port=2
  wires:
  Bus Selector/1 -> Extract Tractor Translation/1(Tractor), Extract Tractor Rotation/1(Tractor)  "<Tractor>"
  Extract Tractor Translation/1(Translation) -> Translation/1
  Vehicle Info/1 -> Bus Selector/1
  Extract Tractor Rotation/1(Rotation) -> Rotation/1

== system PlatooningUsingV2VTestBench/Visualization/Trailer ==
  Vehicle Info : Inport
  Bus Selector1 : BusSelector  OutputSignals=Trailer
  Extract Trailer Rotation : Subsystem
  Extract Trailer Translation : Subsystem
  Translation : Outport
  Rotation : Outport  Port=2
  wires:
  Bus Selector1/1 -> Extract Trailer Rotation/1(Trailer), Extract Trailer Translation/1(Trailer)  "<Trailer>"
  Extract Trailer Rotation/1(Rotation) -> Rotation/1
  Vehicle Info/1 -> Bus Selector1/1
  Extract Trailer Translation/1(Translation) -> Translation/1

== system PlatooningUsingV2VTestBench/Visualization/Trailer1 ==
  Vehicle Info : Inport
  Bus Selector1 : BusSelector  OutputSignals=Trailer
  Extract Trailer Rotation : Subsystem
  Extract Trailer Translation : Subsystem
  Translation : Outport
  Rotation : Outport  Port=2
  wires:
  Bus Selector1/1 -> Extract Trailer Rotation/1(Trailer), Extract Trailer Translation/1(Trailer)  "<Trailer>"
  Extract Trailer Rotation/1(Rotation) -> Rotation/1
  Vehicle Info/1 -> Bus Selector1/1
  Extract Trailer Translation/1(Translation) -> Translation/1

== system PlatooningUsingV2VTestBench/Visualization/Extract Translation and Rotation /Get Translation ==
  Position : Inport
  Constant : Constant  Value=tractor.HitchDistance
  Constant1 : Constant  Value=0  SampleTime=Ts
  Constant2 : Constant  Value=zeros(6,3)  SampleTime=Ts
  Selector : Selector  InputPortWidth=2  IndexOptions=Index vector (dialog)  Indices=1  OutputSizes=1
  Selector1 : Selector  InputPortWidth=2  IndexOptions=Index vector (dialog)  Indices=2  OutputSizes=1
  Sum : Sum  Inputs=-+|
  Transpose : Math  Operator=transpose
  Vector Concatenate : Concatenate  NumInputs=3  Mode=Multidimensional array
  Vector Concatenate1 : Concatenate  Mode=Multidimensional array
  Translation : Outport
  wires:
  Constant2/1 -> Vector Concatenate1/2
  Vector Concatenate/1 -> Transpose/1
  Constant1/1 -> Vector Concatenate/3  "Z"
  Vector Concatenate1/1 -> Translation/1
  Transpose/1 -> Vector Concatenate1/1
  Sum/1 -> Vector Concatenate/1
  Constant/1 -> Sum/1
  Position/1 -> Selector1/1, Selector/1
  Selector/1 -> Sum/2  "X"
  Selector1/1 -> Vector Concatenate/2  "Y"

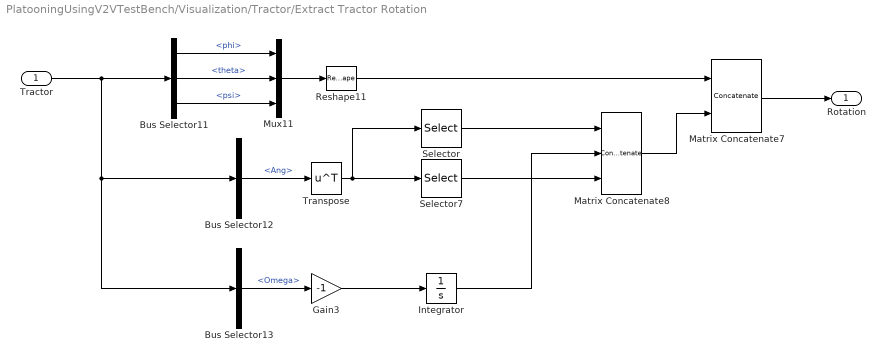
== system PlatooningUsingV2VTestBench/Visualization/Tractor/Extract Tractor Rotation ==
  Tractor : Inport
  Bus Selector11 : BusSelector  OutputSignals=Vehicle.InertFrm.Cg.Ang.phi,Vehicle.InertFrm.Cg.Ang.theta,Vehicle.InertFrm.Cg.Ang.psi
  Bus Selector12 : BusSelector  OutputSignals=Suspension.Whl.Ang
  Bus Selector13 : BusSelector  OutputSignals=Wheels.TireFrame.Omega
  Gain3 : Gain  Gain=-1
  Integrator : Integrator
  Matrix Concatenate7 : Concatenate  Mode=Multidimensional array
  Matrix Concatenate8 : Concatenate  NumInputs=3  Mode=Multidimensional array  ConcatenateDimension=2
  Mux11 : Mux  Inputs=3
  Reshape11 : Reshape  OutputDimensionality=Row vector (2-D)
  Selector : Selector  NumberOfDimensions=2  InputPortWidth=3  IndexOptions=Select all,Index vector (dialog)  Indices=1,1  OutputSizes=1,1
  Selector7 : Selector  NumberOfDimensions=2  InputPortWidth=3  IndexOptions=Select all,Index vector (dialog)  Indices=3,3  OutputSizes=1,1
  Transpose : Math  Operator=transpose
  Rotation : Outport
  wires:
  Transpose/1 -> Selector7/1, Selector/1
  Gain3/1 -> Integrator/1
  Selector7/1 -> Matrix Concatenate8/3
  Bus Selector11/3 -> Mux11/3  "<psi>"
  Bus Selector11/1 -> Mux11/1  "<phi>"
  Bus Selector11/2 -> Mux11/2  "<theta>"
  Reshape11/1 -> Matrix Concatenate7/1
  Selector/1 -> Matrix Concatenate8/1
  Mux11/1 -> Reshape11/1
  Bus Selector12/1 -> Transpose/1  "<Ang>"
  Matrix Concatenate8/1 -> Matrix Concatenate7/2
  Tractor/1 -> Bus Selector13/1, Bus Selector12/1, Bus Selector11/1
  Bus Selector13/1 -> Gain3/1  "<Omega>"
  Integrator/1 -> Matrix Concatenate8/2
  Matrix Concatenate7/1 -> Rotation/1

== system PlatooningUsingV2VTestBench/Visualization/Tractor/Extract Tractor Translation ==
  Tractor : Inport
  Bus Selector3 : BusSelector  OutputSignals=Wheels.TireFrame.z
  Bus Selector8 : BusSelector  OutputSignals=Vehicle.InertFrm.Hitch.Disp.X,Vehicle.InertFrm.Hitch.Disp.Y,Vehicle.InertFrm.Hitch.Disp.Z
  Constant : Constant  Value=tractor.HeightCG-tractor.HitchHeight
  Constant1 : Constant  Value=zeros(6,2)
  Matrix Concatenate1 : Concatenate  Mode=Multidimensional array  ConcatenateDimension=2
  Matrix Concatenate5 : Concatenate  Mode=Multidimensional array
  Mux8 : Mux  Inputs=3
  Reshape : Reshape  OutputDimensionality=Column vector (2-D)
  Reshape8 : Reshape  OutputDimensionality=Row vector (2-D)
  Sum : Sum  Inputs=|+-
  Translation : Outport
  wires:
  Reshape8/1 -> Matrix Concatenate5/1
  Bus Selector8/3 -> Sum/1  "<Z>"
  Sum/1 -> Mux8/3
  Bus Selector8/1 -> Mux8/1  "<X>"
  Mux8/1 -> Reshape8/1
  Matrix Concatenate5/1 -> Translation/1
  Bus Selector8/2 -> Mux8/2  "<Y>"
  Tractor/1 -> Bus Selector8/1, Bus Selector3/1
  Bus Selector3/1 -> Reshape/1  "<z>"
  Reshape/1 -> Matrix Concatenate1/2
  Constant1/1 -> Matrix Concatenate1/1
  Matrix Concatenate1/1 -> Matrix Concatenate5/2
  Constant/1 -> Sum/2
